simulink model "plant_smol"  (R2023b)
settings: Solver=FixedStepAuto  StartTime=0.0  StopTime=SIMTIME  FixedStep=SIMSTEP  RelTol=1e-3
values from neighbouring files (symbols this model uses):
  A = [z33,    eye(3) ... (first row only)    [smol_boat.m]
  B = [z33, inv(M)]'    [smol_boat.m]
  bias = [bias_X;0;0]    [smol_boat.m]
  Bv = [z33, inv(M)]'    [smol_boat.m]
  C = [eye(n_outputs,n_states)]    [smol_boat.m]
  x0 = zeros(n_states,1)    [smol_boat.m]
settings Model: Creator=X20  LastModifiedBy=Lorenzo-Desk
settings DataIOCC: ReturnWorkspaceOutputs=off

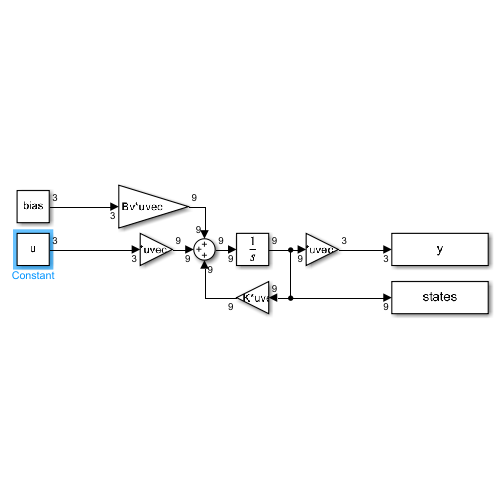
[thumbnail: Simulink's stored preview of the top-level diagram]
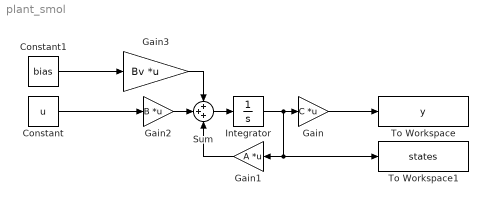
== system plant_smol ==
  Constant : Constant  Value=u
  Constant1 : Constant  Value=bias
  Gain : Gain  Gain=C  Multiplication=Matrix(K*u) (u vector)
  Gain1 : Gain  Gain=A  Multiplication=Matrix(K*u) (u vector)
  Gain2 : Gain  Gain=B  Multiplication=Matrix(K*u) (u vector)
  Gain3 : Gain  Gain=Bv  Multiplication=Matrix(K*u) (u vector)
  Integrator : Integrator  InitialCondition=x0
  Sum : Sum  Inputs=+++
  To Workspace : ToWorkspace  VariableName=y  SaveFormat=Timeseries  SampleTime=-1
  To Workspace1 : ToWorkspace  VariableName=states  SaveFormat=Timeseries  SampleTime=-1
  wires:
  Sum/1 -> Integrator/1
  Gain1/1 -> Sum/3
  Constant/1 -> Gain2/1
  Gain/1 -> To Workspace/1
  Gain2/1 -> Sum/2
  Gain3/1 -> Sum/1
  Integrator/1 -> Gain/1, Gain1/1, To Workspace1/1
  Constant1/1 -> Gain3/1
